simulink model "chap2_6sim"  (R2016a)
settings: Solver=VariableStepAuto  StartTime=0.0  StopTime=10.0  RelTol=1e-3
values from neighbouring files (symbols this model uses):
  K = 10    [Chap2_6int.m]    (also in chap2_3.m = 1)
  tol = 1.0    (= 1)    [Chap2_6int.m]    (also in Chap2_9.m = 80; chap2_3.m = 80)
undefined symbols (not defined in the file): Kd, Kp
settings Model: Creator=zhanghankui  LastModifiedBy=zhanghankui

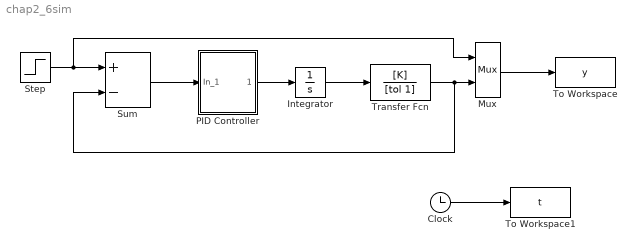
== system chap2_6sim ==
  Clock : Clock
  Integrator : Integrator
  Mux : Mux  Inputs=2
  PID Controller : Subsystem  mask(PID Controller){P=Kp, I=0, D=Kd}
      mask prompts: P "Proportional:"; I "Integral:"; D "Derivative:"
      mask help:
      | Enter expressions for proportional, integral, and derivative terms.
      | P+I/s+Ds
      mask Help: This block implements a PID controller where parameters are entered for the Proportional, Integral and Derivative terms. Unmask this block to see how it works. The derivative term is implemented using a true derivative block.
      mask Display: disp('PID')
  Step : Step  Time=0  SampleTime=0
  Sum : Sum  Inputs=+-
  To Workspace : ToWorkspace  VariableName=y  SampleTime=-1
      settings: Save2DSignal=2-D array (concatenate along first dimension)
  To Workspace1 : ToWorkspace  VariableName=t  SampleTime=-1
      settings: Save2DSignal=2-D array (concatenate along first dimension)
  Transfer Fcn : TransferFcn  Numerator=[K]  Denominator=[tol 1]
  wires:
  Step/1 -> Mux/1, Sum/1
  Sum/1 -> PID Controller/1(In_1)
  PID Controller/1(Out_1) -> Integrator/1
  Integrator/1 -> Transfer Fcn/1
  Mux/1 -> To Workspace/1
  Transfer Fcn/1 -> Sum/2, Mux/2
  Clock/1 -> To Workspace1/1

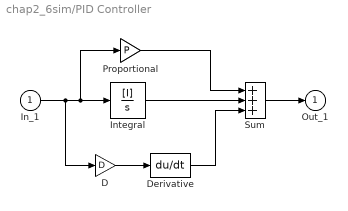
== system chap2_6sim/PID Controller ==
  In_1 : Inport
  D : Gain  Gain=D  SaturateOnIntegerOverflow=on  OutDataTypeStr=Inherit: Same as input  ParamDataTypeStr=Inherit: Same as input
  Derivative : Derivative
  Integral : TransferFcn  Numerator=[I]  Denominator=[1 0]
  Proportional : Gain  Gain=P  SaturateOnIntegerOverflow=on  OutDataTypeStr=Inherit: Same as input  ParamDataTypeStr=Inherit: Same as input
  Sum : Sum  Inputs=+++  SaturateOnIntegerOverflow=on  InputSameDT=on  OutDataTypeStr=Inherit: Same as first input
  Out_1 : Outport  InitialOutput=0
  wires:
  D/1 -> Derivative/1
  Sum/1 -> Out_1/1
  In_1/1 -> D/1, Proportional/1, Integral/1
  Integral/1 -> Sum/2
  Proportional/1 -> Sum/1
  Derivative/1 -> Sum/3
